simulink model "es1"  (R2018a)
settings: Solver=VariableStepAuto  StartTime=0.0  StopTime=10.0  RelTol=1e-3
values from neighbouring files (symbols this model uses):
  B = 0.02    [data.m]
  J = 0.1    [data.m]
  K_a = 10    [data.m]
  K_m = 0.5    [data.m]
  L_a = 6e-3    (= 0.006)    [data.m]
  R_a = 1    [data.m]
settings Model: Creator=Ale  LastModifiedBy=Ale

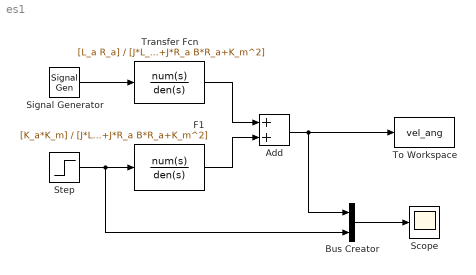
== system es1 ==
  Add : Sum
  Bus Creator : BusCreator  Inputs=2
  F1 : TransferFcn  Numerator=[K_a*K_m]  Denominator=[J*L_a B*L_a+J*R_a B*R_a+K_m^2]
  Scope : Scope
  Signal Generator : SignalGenerator  WaveForm=square  Amplitude=0.05  Frequency=0.1
  Step : Step  Time=0  After=(B*R_a+K_m^2)/(K_a*K_m)  SampleTime=0
  To Workspace : ToWorkspace  VariableName=vel_ang  SaveFormat=Timeseries  SampleTime=-1
  Transfer Fcn : TransferFcn  Numerator=[L_a R_a]  Denominator=[J*L_a B*L_a+J*R_a B*R_a+K_m^2]
  wires:
  Step/1 -> Bus Creator/2, F1/1
  Signal Generator/1 -> Transfer Fcn/1
  Transfer Fcn/1 -> Add/1
  F1/1 -> Add/2
  Add/1 -> Bus Creator/1, To Workspace/1
  Bus Creator/1 -> Scope/1
